simulink model "cartpole_MOE_2019a"  (R2019a)
settings: Solver=ode1  StartTime=0.0  StopTime=inf  FixedStep=0.001  RelTol=1e-3
values from neighbouring files (symbols this model uses):
  binb1 = reshape(psi(binLayerRanges(1, 3):binLayerRanges(1, 4)), binLayers(2), 1)    [main.m]
  binb2 = reshape(psi(binLayerRanges(2, 3):binLayerRanges(2, 4)), binLayers(3), 1)    [main.m]
  binb3 = reshape(psi(binLayerRanges(3, 3):binLayerRanges(3, 4)), binLayers(4), 1)    [main.m]
  binW1 = reshape(psi(binLayerRanges(1, 1):binLayerRanges(1, 2)), binLayers(2), binLayers(1))    [main.m]
  binW2 = reshape(psi(binLayerRanges(2, 1):binLayerRanges(2, 2)), binLayers(3), binLayers(2))    [main.m]
  binW3 = reshape(psi(binLayerRanges(3, 1):binLayerRanges(3, 2)), binLayers(4), binLayers(3))    [main.m]
  control1b1 = reshape(theta1(control1LayerRanges(1, 3):control1LayerRanges(1, 4)), control1Layers(2), 1)    [main.m]
  control1b2 = reshape(theta1(control1LayerRanges(2, 3):control1LayerRanges(2, 4)), control1Layers(3), 1)    [main.m]
  control1b3 = reshape(theta1(control1LayerRanges(3, 3):control1LayerRanges(3, 4)), control1Layers(4), 1)    [main.m]
  control1W1 = reshape(theta1(control1LayerRanges(1, 1):control1LayerRanges(1, 2)), control1Layers(2), control1Layers(1))    [main.m]
  control1W2 = reshape(theta1(control1LayerRanges(2, 1):control1LayerRanges(2, 2)), control1Layers(3), control1Layers(2))    [main.m]
  control1W3 = reshape(theta1(control1LayerRanges(3, 1):control1LayerRanges(3, 2)), control1Layers(4), control1Layers(3))    [main.m]
  control2b1 = reshape(theta2(control2LayerRanges(1, 3):control2LayerRanges(1, 4)), control2Layers(2), 1)    [main.m]
  control2b2 = reshape(theta2(control2LayerRanges(2, 3):control2LayerRanges(2, 4)), control2Layers(3), 1)    [main.m]
  control2b3 = reshape(theta2(control2LayerRanges(3, 3):control2LayerRanges(3, 4)), control2Layers(4), 1)    [main.m]
  control2W1 = reshape(theta2(control2LayerRanges(1, 1):control2LayerRanges(1, 2)), control2Layers(2), control2Layers(1))    [main.m]
  control2W2 = reshape(theta2(control2LayerRanges(2, 1):control2LayerRanges(2, 2)), control2Layers(3), control2Layers(2))    [main.m]
  control2W3 = reshape(theta2(control2LayerRanges(3, 1):control2LayerRanges(3, 2)), control2Layers(4), control2Layers(3))    [main.m]
  control3b1 = reshape(theta3(control3LayerRanges(1, 3):control3LayerRanges(1, 4)), control3Layers(2), 1)    [main.m]
  control3b2 = reshape(theta3(control3LayerRanges(2, 3):control3LayerRanges(2, 4)), control3Layers(3), 1)    [main.m]
  control3b3 = reshape(theta3(control3LayerRanges(3, 3):control3LayerRanges(3, 4)), control3Layers(4), 1)    [main.m]
  control3W1 = reshape(theta3(control3LayerRanges(1, 1):control3LayerRanges(1, 2)), control3Layers(2), control3Layers(1))    [main.m]
  control3W2 = reshape(theta3(control3LayerRanges(2, 1):control3LayerRanges(2, 2)), control3Layers(3), control3Layers(2))    [main.m]
  control3W3 = reshape(theta3(control3LayerRanges(3, 1):control3LayerRanges(3, 2)), control3Layers(4), control3Layers(3))    [main.m]
  Fmax = 4.5    [main.m]
  lqr_gains = [-0.707107;  25.8856; -3.51898; 4.49824]    [main.m]
undefined symbols (not defined in the file or in its folder): af, bf, HIL, Kt, Nenc, qc_get_step_size, R, r_enc, rg, rm, T, Vmax
libraries: quarc_library x3
settings Model: SimulationMode=external  ExtModeTrigDuration=5000  Creator=johnchiasson  LastModifiedBy=NardosAshenafi
settings SolverCC: PositivePriorityOrder=on
settings DataIOCC: LimitDataPoints=on  SaveFormat=Array  ReturnWorkspaceOutputs=off
settings OptimizationCC: LifeSpan=inf
settings DebuggingCC: SFUnexpectedBacktrackingDiag=warning  SFNoUnconditionalDefaultTransitionDiag=warning  SFExecutionAtInitializationDiag=none  ArithmeticOperatorsInVariantConditions=warning
settings HardwareCC: ProdBitPerPointer=32  ProdBitPerSizeT=32  ProdBitPerPtrDiffT=32  ProdLargestAtomicFloat=None  ProdIntDivRoundTo=Undefined  ProdEndianess=Unspecified  ProdWordSize=32  ProdHWDeviceType=32-bit Generic
settings ModelReferenceCC: PropagateSignalLabelsOutOfModel=off
settings SFSimCC: SimUseLocalCustomCode=off
settings RTWCC: SystemTargetFile=quarc_win64.tlc  TemplateMakefile=quarc_default_tmf  Description=QUARC Win64 Target  RTWUseLocalCustomCode=off
settings CodeAppCC: StateflowObjectComments=on
settings STFCustomTargetCC: TargetPreCompLibLocation=C:\PROGRA~3\QUARC\lib\2019a\win64\release  ConcurrentExecutionCompliant=on  SystemTargetFile=quarc_win64.tlc
settings GRTTargetCC: TargetPreCompLibLocation=C:\PROGRA~3\QUARC\lib\2019a\win64\release  TargetLangStandard=C89/C90 (ANSI)  ParMdlRefBuildCompliant=off  CompOptLevelCompliant=off  CombineOutputUpdateFcns=off  MatFileLogging=off  CPPClassGenCompliant=off  GRTInterface=on  UseToolchainInfoCompliant=off  ExtMode=on  ExtModeMexFile=quarc_comm
settings ConfigComp: CovMetricSettings=dw  CovSaveCumulativeToWorkspaceVar=on  CovSaveSingleToWorkspaceVar=on  CovExternalEMLEnable=off

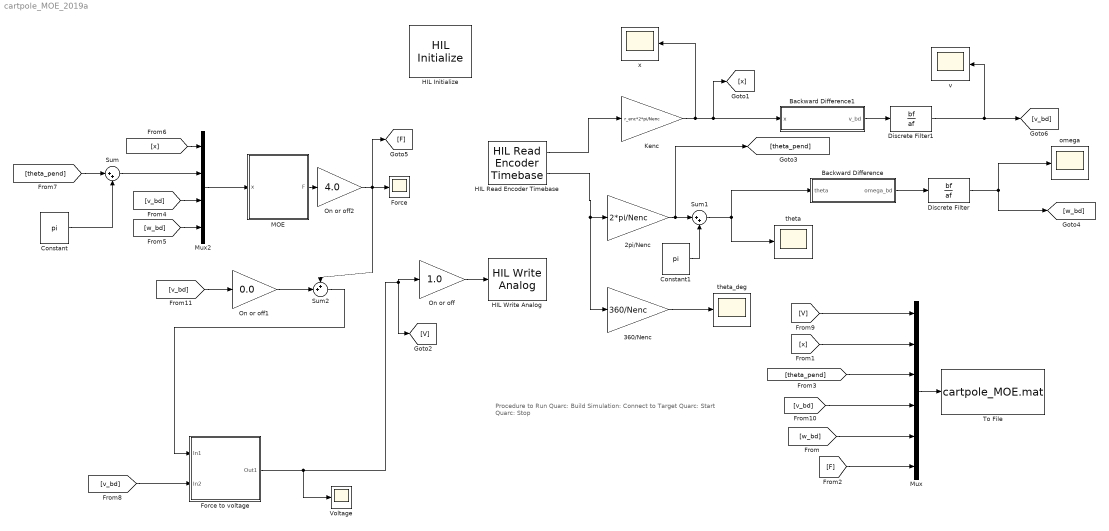
== system cartpole_MOE_2019a ==
  note: Procedure to Run
      |
      | Quarc: Build
      | Simulation: Connect to Target
      | Quarc: Start
      | Quarc: Stop
  2pi/Nenc : Gain  Gain=2*pi/Nenc
  360/Nenc : Gain  Gain=360/Nenc
  Backward Difference : Subsystem
  Backward Difference1 : Subsystem
  Constant : Constant  Value=pi
  Constant1 : Constant  Value=pi
  Discrete Filter : DiscreteFilter  Numerator=bf  Denominator=af
  Discrete Filter1 : DiscreteFilter  Numerator=bf  Denominator=af
  Force : Scope
  Force to voltage : Subsystem
  HIL Initialize : quarc_library/Data Acquisition/Generic/Configuration/HIL Initialize  Priority=-99  object_name=HIL-1  board_type=q2_usb  board_number=0  board_options=d0=digital;d1=digital;led=auto;update_rate=normal;decimation=1  exclusive=off  active=off  hardware_clocks=[0]  clock_modes=[]  initial_clock_frequencies=[]  set_clock_params_at_start=off  set_clock_params_at_switch_in=off  set_clock_frequencies_at_start=off  set_clock_frequencies_at_switch_in=off  analog_input_channels=[0:1]  analog_input_configurations=[]  analog_input_maximums=10  analog_input_minimums=-10  set_analog_input_params_at_start=on  set_analog_input_params_at_switch_in=off  analog_output_channels=[0:1]  analog_output_maximums=10  analog_output_minimums=-10  initial_analog_outputs=[0]  final_analog_outputs=[0]  watchdog_analog_outputs=0  set_analog_output_params_at_start=on  set_analog_output_params_at_switch_in=off  set_analog_outputs_at_start=on  set_analog_outputs_at_switch_in=off  set_analog_outputs_at_terminate=on  set_analog_outputs_at_switch_out=off  set_analog_outputs_on_watchdog=off  digital_input_channels=[]  digital_output_channels=[]  digital_output_configuration=[]  initial_digital_outputs=[1]  final_digital_outputs=[1]  watchdog_digital_outputs=[1]  set_digital_output_params_at_start=off  set_digital_output_params_at_switch_in=off  set_digital_outputs_at_start=on  set_digital_outputs_at_switch_in=off  set_digital_outputs_at_terminate=on  set_digital_outputs_at_switch_out=off  set_digital_outputs_on_watchdog=off  encoder_channels=[0:1]  quadrature=[4]  encoder_filter_frequency=[]  initial_encoder_counts=[0]  set_encoder_params_at_start=on  set_encoder_params_at_switch_in=off  set_encoder_counts_at_start=on  set_encoder_counts_at_switch_in=off  pwm_channels=[]  pwm_modes=[0]  pwm_frequency=1/0.020  pwm_configuration=[]  pwm_alignment=[]  pwm_polarity=[]  pwm_leading_deadband=[]  pwm_trailing_deadband=[]  initial_pwm_outputs=[0]  final_pwm_outputs=[0]  watchdog_pwm_outputs=[0]  set_pwm_params_at_start=on  set_pwm_params_at_switch_in=off  set_pwm_outputs_at_start=on  set_pwm_outputs_at_switch_in=off  set_pwm_outputs_at_terminate=on  set_pwm_outputs_at_switch_out=off  set_pwm_outputs_on_watchdog=off  other_output_channels=[]  initial_other_outputs=[]  final_other_outputs=[]  watchdog_other_outputs=[]  set_other_outputs_at_start=off  set_other_outputs_at_switch_in=off  set_other_outputs_at_terminate=off  set_other_outputs_at_switch_out=off  set_other_outputs_on_watchdog=off
  HIL Read Encoder Timebase : quarc_library/Data Acquisition/Generic/Timebases/HIL Read Encoder Timebase  object_name=HIL-1  clock=0  channels=[0:1]  samples_in_buffer=max(ceil(1/qc_get_step_size), 1)  active=on  vector_output=off  data_type_mode=Inherit via back propagation  data_type=double
  HIL Write Analog : quarc_library/Data Acquisition/Generic/Immediate I//O/HIL Write Analog  object_name=HIL-1  channels=0  sample_time=-1  active=off  vector_input=off
  Kenc : Gain  Gain=r_enc*2*pi/Nenc
  MOE : Subsystem
  Mux : Mux  Inputs=6
  Mux2 : Mux
  On or off : Gain  Gain=1.0
  On or off1 : Gain  Gain=0.0
  On or off2 : Gain  Gain=4.0
  Sum : Sum  Inputs=|++
  Sum1 : Sum  Inputs=|++
  Sum2 : Sum  Inputs=++|
  To File : ToFile  Filename=cartpole_MOE.mat  MatrixName=cart_data  SampleTime=T
  Voltage : Scope
  omega : Scope
  theta : Scope
  theta_deg : Scope
  v : Scope
  x : Scope
  wires:
  HIL Read Encoder Timebase/1 -> Kenc/1
  HIL Read Encoder Timebase/2 -> 360/Nenc/1, 2pi/Nenc/1
  Kenc/1 -> x/1, Backward Difference1/1(x), [x]
  360/Nenc/1 -> theta_deg/1
  Mux/1 -> To File/1
  [V] -> Mux/1
  [x] -> Mux/2
  [theta_pend] -> Mux/3
  [v_bd] -> Mux/4
  Force to voltage/1(Out1) -> Voltage/1, [V], On or off/1
  [x] -> Mux2/1
  [v_bd] -> Mux2/3
  Mux2/1 -> MOE/1(x)
  [v_bd] -> Force to voltage/2(In2)
  [w_bd] -> Mux2/4
  On or off/1 -> HIL Write Analog/1
  [w_bd] -> Mux/5
  [F] -> Mux/6
  Backward Difference/1(omega_bd) -> Discrete Filter/1
  Discrete Filter/1 -> [w_bd], omega/1
  Backward Difference1/1(v_bd) -> Discrete Filter1/1
  Discrete Filter1/1 -> v/1, [v_bd]
  [theta_pend] -> Sum/1
  Constant/1 -> Sum/2
  Sum/1 -> Mux2/2
  2pi/Nenc/1 -> [theta_pend], Sum1/1
  Constant1/1 -> Sum1/2
  Sum1/1 -> Backward Difference/1(theta), theta/1
  [v_bd] -> On or off1/1
  On or off1/1 -> Sum2/2
  Sum2/1 -> Force to voltage/1(In1)
  On or off2/1 -> Sum2/1, [F], Force/1
  MOE/1(F) -> On or off2/1

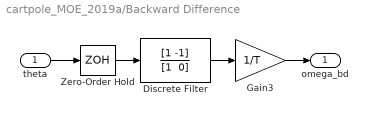
== system cartpole_MOE_2019a/Backward Difference ==
  theta : Inport
  Discrete Filter : DiscreteFilter  Numerator=[1 -1]  Denominator="[1  0]"
  Gain3 : Gain  Gain=1/T  SaturateOnIntegerOverflow=on  OutDataTypeStr=Inherit: Same as input  ParamDataTypeStr=Inherit: Same as input
  Zero-Order Hold : ZeroOrderHold  SampleTime=T
  omega_bd : Outport
  wires:
  Discrete Filter/1 -> Gain3/1
  Gain3/1 -> omega_bd/1
  Zero-Order Hold/1 -> Discrete Filter/1
  theta/1 -> Zero-Order Hold/1

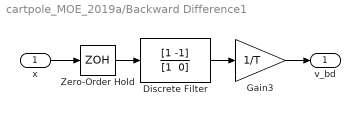
== system cartpole_MOE_2019a/Backward Difference1 ==
  x : Inport
  Discrete Filter : DiscreteFilter  Numerator=[1 -1]  Denominator="[1  0]"
  Gain3 : Gain  Gain=1/T  SaturateOnIntegerOverflow=on  OutDataTypeStr=Inherit: Same as input  ParamDataTypeStr=Inherit: Same as input
  Zero-Order Hold : ZeroOrderHold  SampleTime=T
  v_bd : Outport
  wires:
  Discrete Filter/1 -> Gain3/1
  Gain3/1 -> v_bd/1
  Zero-Order Hold/1 -> Discrete Filter/1
  x/1 -> Zero-Order Hold/1

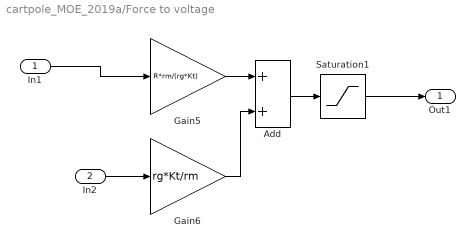
== system cartpole_MOE_2019a/Force to voltage ==
  In1 : Inport
  In2 : Inport  Port=2
  Add : Sum
  Gain5 : Gain  Gain=R*rm/(rg*Kt)  SaturateOnIntegerOverflow=on  OutDataTypeStr=Inherit: Same as input  ParamDataTypeStr=Inherit: Same as input
  Gain6 : Gain  Gain=rg*Kt/rm  SaturateOnIntegerOverflow=on  OutDataTypeStr=Inherit: Same as input  ParamDataTypeStr=Inherit: Same as input
  Saturation1 : Saturate  UpperLimit=Vmax  LowerLimit=-Vmax
  Out1 : Outport  VectorParamsAs1DForOutWhenUnconnected=on
  wires:
  Add/1 -> Saturation1/1
  Gain5/1 -> Add/1
  Saturation1/1 -> Out1/1
  In1/1 -> Gain5/1
  Gain6/1 -> Add/2
  In2/1 -> Gain6/1

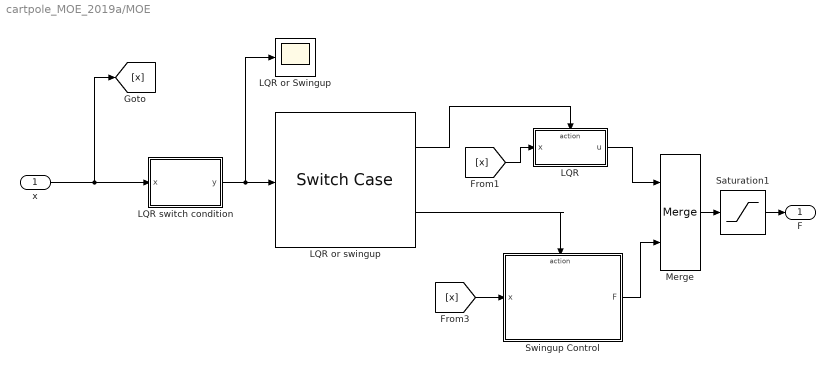
== system cartpole_MOE_2019a/MOE ==
  x : Inport
  LQR : Subsystem  TreatAsAtomicUnit=on
  LQR or Swingup : Scope
  LQR or swingup : SwitchCase  CaseConditions={1, 2}  ShowDefaultCase=off
  LQR switch condition : MATLAB Function  TreatAsAtomicUnit=on
  Merge : Merge
  Saturation1 : Saturate  UpperLimit=Fmax  LowerLimit=-Fmax
  Swingup Control : Subsystem  TreatAsAtomicUnit=on
  F : Outport
  wires:
  x/1 -> LQR switch condition/1(x), [x]
  LQR or swingup/2 -> Swingup Control/Action
  [x] -> Swingup Control/1(x)
  Merge/1 -> Saturation1/1
  Swingup Control/1(F) -> Merge/2
  LQR or swingup/1 -> LQR/Action
  [x] -> LQR/1(x)
  LQR/1(u) -> Merge/1
  LQR switch condition/1(y) -> LQR or Swingup/1, LQR or swingup/1
  Saturation1/1 -> F/1

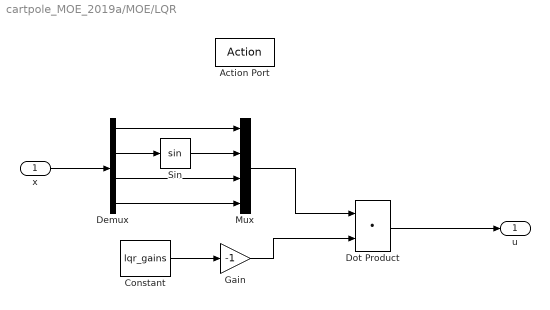
== system cartpole_MOE_2019a/MOE/LQR ==
  x : Inport
  Action Port : ActionPort  ActionPortLabel=case [ 1 ]:
  Constant : Constant  Value=lqr_gains
  Demux : Demux
  Dot Product : DotProduct  InputSameDT=on  OutDataTypeStr=Inherit: Inherit via internal rule
  Gain : Gain  Gain=-1
  Mux : Mux
  Sin : Trigonometry
  u : Outport  VectorParamsAs1DForOutWhenUnconnected=on
  wires:
  x/1 -> Demux/1
  Dot Product/1 -> u/1
  Constant/1 -> Gain/1
  Gain/1 -> Dot Product/2
  Demux/1 -> Mux/1
  Demux/2 -> Sin/1
  Sin/1 -> Mux/2
  Demux/3 -> Mux/3
  Demux/4 -> Mux/4
  Mux/1 -> Dot Product/1

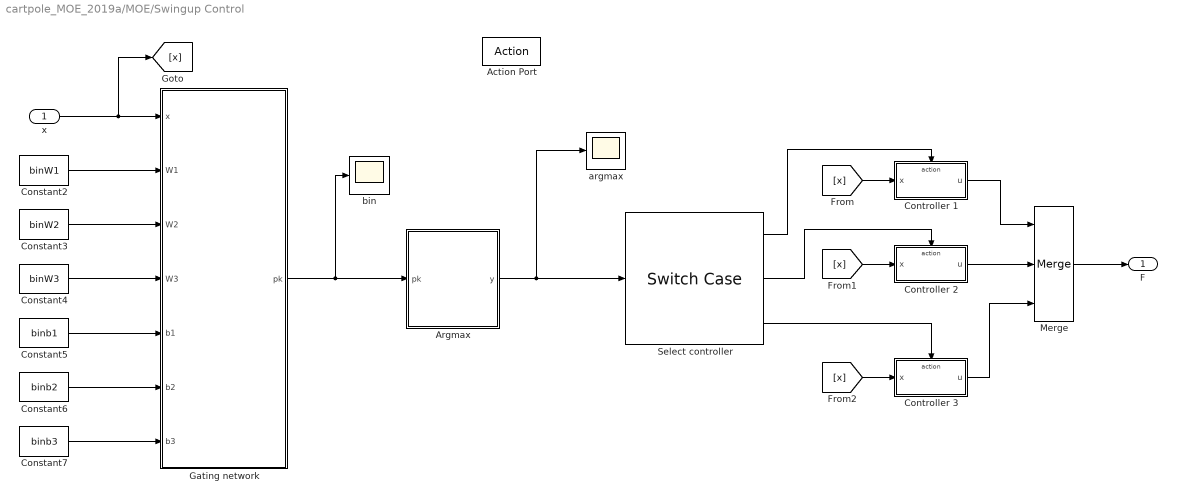
== system cartpole_MOE_2019a/MOE/Swingup Control ==
  x : Inport
  Action Port : ActionPort  ActionPortLabel=case [ 2 ]:
  Argmax : MATLAB Function  TreatAsAtomicUnit=on
  Constant2 : Constant  Value=binW1
  Constant3 : Constant  Value=binW2
  Constant4 : Constant  Value=binW3
  Constant5 : Constant  Value=binb1
  Constant6 : Constant  Value=binb2
  Constant7 : Constant  Value=binb3
  Controller 1 : Subsystem  TreatAsAtomicUnit=on
  Controller 2 : Subsystem  TreatAsAtomicUnit=on
  Controller 3 : Subsystem  TreatAsAtomicUnit=on
  Gating network : MATLAB Function  TreatAsAtomicUnit=on
  Merge : Merge  Inputs=3
  Select controller : SwitchCase  CaseConditions={1, 2, 3}  ShowDefaultCase=off
  argmax : Scope
  bin : Scope
  F : Outport
  wires:
  [x] -> Controller 3/1(x)
  Constant2/1 -> Gating network/2(W1)
  Select controller/3 -> Controller 3/Action
  Gating network/1(pk) -> Argmax/1(pk), bin/1
  Controller 1/1(u) -> Merge/1
  [x] -> Controller 2/1(x)
  Constant6/1 -> Gating network/6(b2)
  Select controller/2 -> Controller 2/Action
  Constant3/1 -> Gating network/3(W2)
  [x] -> Controller 1/1(x)
  Constant5/1 -> Gating network/5(b1)
  Controller 3/1(u) -> Merge/3
  Constant4/1 -> Gating network/4(W3)
  Select controller/1 -> Controller 1/Action
  Controller 2/1(u) -> Merge/2
  Constant7/1 -> Gating network/7(b3)
  Argmax/1(y) -> argmax/1, Select controller/1
  Merge/1 -> F/1
  x/1 -> [x], Gating network/1(x)

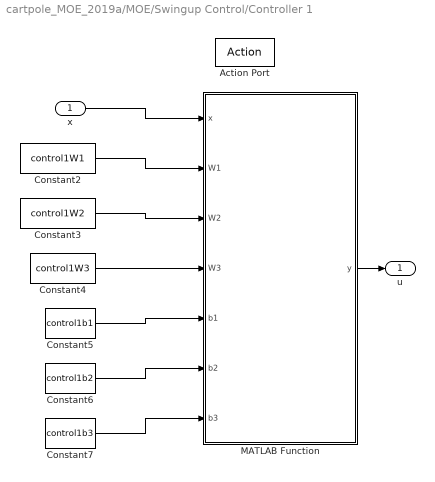
== system cartpole_MOE_2019a/MOE/Swingup Control/Controller 1 ==
  x : Inport
  Action Port : ActionPort  ActionPortLabel=case [ 1 ]:
  Constant2 : Constant  Value=control1W1
  Constant3 : Constant  Value=control1W2
  Constant4 : Constant  Value=control1W3  VectorParams1D=off
  Constant5 : Constant  Value=control1b1
  Constant6 : Constant  Value=control1b2
  Constant7 : Constant  Value=control1b3
  MATLAB Function : MATLAB Function  TreatAsAtomicUnit=on
  u : Outport  VectorParamsAs1DForOutWhenUnconnected=on
  wires:
  Constant2/1 -> MATLAB Function/2(W1)
  Constant5/1 -> MATLAB Function/5(b1)
  Constant7/1 -> MATLAB Function/7(b3)
  Constant6/1 -> MATLAB Function/6(b2)
  Constant4/1 -> MATLAB Function/4(W3)
  Constant3/1 -> MATLAB Function/3(W2)
  x/1 -> MATLAB Function/1(x)
  MATLAB Function/1(y) -> u/1

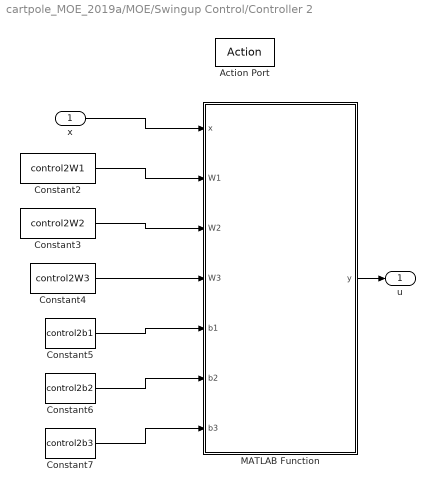
== system cartpole_MOE_2019a/MOE/Swingup Control/Controller 2 ==
  x : Inport
  Action Port : ActionPort  ActionPortLabel=case [ 2 ]:
  Constant2 : Constant  Value=control2W1
  Constant3 : Constant  Value=control2W2
  Constant4 : Constant  Value=control2W3  VectorParams1D=off
  Constant5 : Constant  Value=control2b1
  Constant6 : Constant  Value=control2b2
  Constant7 : Constant  Value=control2b3
  MATLAB Function : MATLAB Function  TreatAsAtomicUnit=on
  u : Outport  VectorParamsAs1DForOutWhenUnconnected=on
  wires:
  Constant7/1 -> MATLAB Function/7(b3)
  Constant2/1 -> MATLAB Function/2(W1)
  Constant3/1 -> MATLAB Function/3(W2)
  Constant4/1 -> MATLAB Function/4(W3)
  MATLAB Function/1(y) -> u/1
  x/1 -> MATLAB Function/1(x)
  Constant6/1 -> MATLAB Function/6(b2)
  Constant5/1 -> MATLAB Function/5(b1)

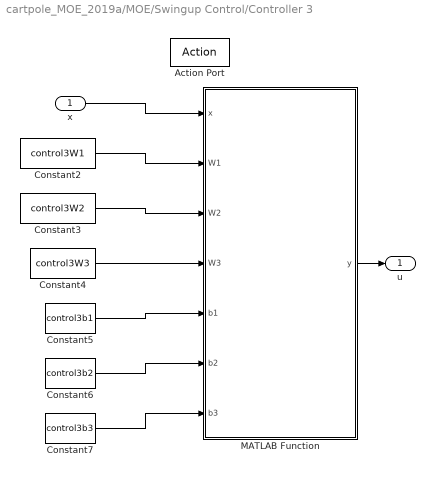
== system cartpole_MOE_2019a/MOE/Swingup Control/Controller 3 ==
  x : Inport
  Action Port : ActionPort  ActionPortLabel=case [ 3 ]:
  Constant2 : Constant  Value=control3W1
  Constant3 : Constant  Value=control3W2
  Constant4 : Constant  Value=control3W3  VectorParams1D=off
  Constant5 : Constant  Value=control3b1
  Constant6 : Constant  Value=control3b2
  Constant7 : Constant  Value=control3b3
  MATLAB Function : MATLAB Function  TreatAsAtomicUnit=on
  u : Outport  VectorParamsAs1DForOutWhenUnconnected=on
  wires:
  Constant7/1 -> MATLAB Function/7(b3)
  Constant2/1 -> MATLAB Function/2(W1)
  Constant3/1 -> MATLAB Function/3(W2)
  Constant4/1 -> MATLAB Function/4(W3)
  MATLAB Function/1(y) -> u/1
  x/1 -> MATLAB Function/1(x)
  Constant6/1 -> MATLAB Function/6(b2)
  Constant5/1 -> MATLAB Function/5(b1)

== matlab function cartpole_MOE_2019a/MOE/LQR switch condition ==
  data: x input; y output
function y = fcn(x)
    z = [x(1); cos(x(2)); sin(x(2)); x(3); x(4)];
    if ((1.0 - z(2)) <= (1.0 - cosd(15)) && (abs(z(5)) <= 1.5))
        y = 1;      %use LQR
    else
        y = 2;      %use swingup control
    end

== matlab function cartpole_MOE_2019a/MOE/Swingup Control/Argmax ==
  data: pk input; y output
function y = fcn(pk)
    maxindex = 1;
    for i = 1:length(pk)-1
       if pk(i+1) > pk(maxindex)
           maxindex = i+1;
       end
    end
y = maxindex;

== matlab function cartpole_MOE_2019a/MOE/Swingup Control/Gating network ==
  data: x input; W1 input; pk output; W2 input; W3 input; b1 input; b2 input; b3 input
function pk = fcn(x, W1, W2, W3, b1, b2, b3)

    z0 = [x(1); cos(x(2)); sin(x(2)); x(3); x(4)];
    z1 = elu(W1*z0 + b1);
    z2 = elu(W2*z1 + b2);
    z3 = W3*z2 + b3;
    pk = softmax(z3);
    
end
    
function y = softmax(x)
    y = zeros(length(x));
    for i =1:length(x)
        y(i) = exp(x(i))/sum(exp(x));
    end
end

== matlab function cartpole_MOE_2019a/MOE/Swingup Control/Controller 1/MATLAB Function ==
  data: x input; y output; W1 input; W2 input; W3 input; b1 input; b2 input; b3 input
function y = fcn(x, W1, W2, W3, b1, b2, b3)
    z0 = [x(1); cos(x(2)); sin(x(2)); x(3); x(4)];
    z1 = elu(W1*z0 + b1);
    z2 = elu(W2*z1 + b2);
    z3 = W3*z2 + b3;
y = z3;

== matlab function cartpole_MOE_2019a/MOE/Swingup Control/Controller 2/MATLAB Function ==
  data: x input; y output; W1 input; W2 input; W3 input; b1 input; b2 input; b3 input
function y = fcn(x, W1, W2, W3, b1, b2, b3)
    z0 = [x(1); cos(x(2)); sin(x(2)); x(3); x(4)];
    z1 = elu(W1*z0 + b1);
    z2 = elu(W2*z1 + b2);
    z3 = W3*z2 + b3;
y = z3;

== matlab function cartpole_MOE_2019a/MOE/Swingup Control/Controller 3/MATLAB Function ==
  data: x input; y output; W1 input; W2 input; W3 input; b1 input; b2 input; b3 input
function y = fcn(x, W1, W2, W3, b1, b2, b3)
    z0 = [x(1); cos(x(2)); sin(x(2)); x(3); x(4)];
    z1 = elu(W1*z0 + b1);
    z2 = elu(W2*z1 + b2);
    z3 = W3*z2 + b3;
y = z3;
